simulink model "fft_dsp_lib"  (R2021a)
settings: Solver=VariableStepAuto  StartTime=0.0  StopTime=1  RelTol=1e-3
undefined symbols (not defined in the file): xc7vx485tffg1157
libraries: simulink x1, dspxfrm3 x1, vmcUtilities x1, dspsrcs4 x1, aieUtilities x1, aieDSP x1
settings Model: Creator=abehbood  LastModifiedBy=abehbood
settings SolverCC: AlgebraicLoopSolver=TrustRegion
settings DebuggingCC: SFMachineParentedDataDiag=warning
settings HardwareCC: ProdBitPerPointer=32  ProdBitPerSizeT=32  ProdBitPerPtrDiffT=32  ProdLargestAtomicFloat=None  ProdIntDivRoundTo=Undefined  ProdEndianess=Unspecified  ProdWordSize=32  ProdHWDeviceType=ASIC/FPGA->ASIC/FPGA  TargetBitPerLong=64  TargetBitPerPointer=64  TargetBitPerSizeT=64  TargetBitPerPtrDiffT=64  TargetLongLongMode=on  TargetIntDivRoundTo=Zero  TargetEndianess=LittleEndian  TargetWordSize=64  TargetHWDeviceType=Custom Processor->MATLAB Host Computer  ProdEqTarget=off

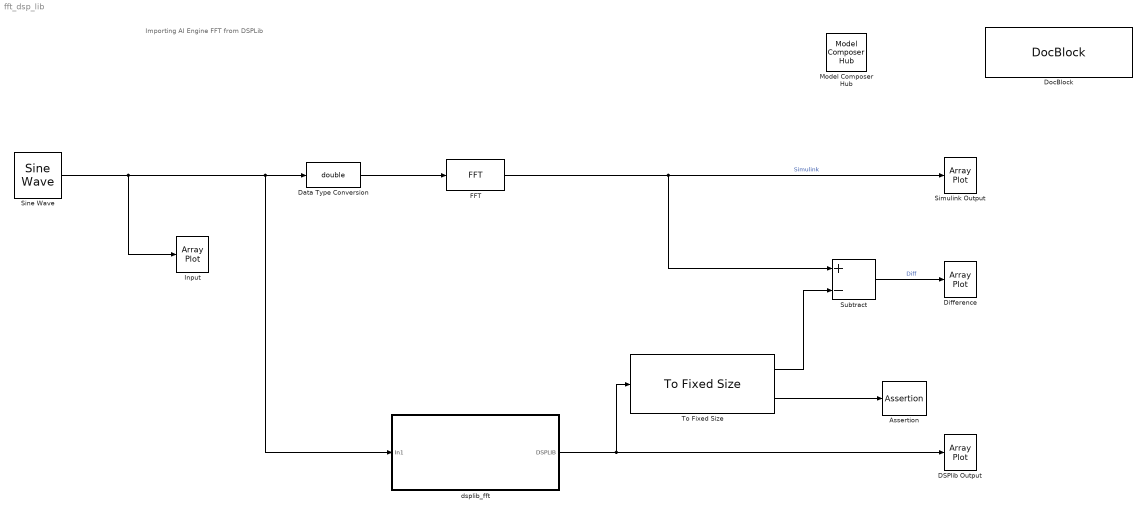
== system fft_dsp_lib ==
  note: Importing AI Engine FFT from DSPLib
  Assertion : Assertion
  DSPlib Output : ArrayPlot  WindowPosition=[34.000000,414.000000,816.000000,354.000000,]  Visible=on  AxesScaling=Manual  YLimits=[-23969.1,17302.1]  ShowLegend=on  DefaultConfigurationName=dsp.scopes.ArrayPlotBlockSpecification
  Data Type Conversion : DataTypeConversion  OutDataTypeStr=double
  Difference : ArrayPlot  WindowPosition=[4.000000,48.000000,780.000000,336.000000,]  Visible=on  AxesScaling=Manual  Title=Difference between AI Engine and Simulink  YLimits=[-461.936,415.69]  ShowLegend=on  DefaultConfigurationName=dsp.scopes.ArrayPlotBlockSpecification
  DocBlock : simulink/Model-Wide Utilities/DocBlock  DocumentType=Text  mask(DocBlock){}
      content=|
      | ///////////////////////////////////////////////////////////////////////////
      | // Copyright 2021 Xilinx
      | //
      | // Licensed under the Apache License, Version 2.0 (the "License");
      | // you may not use this file except in compliance with the License.
      | // You may obtain a copy of the License at
      | //
      | // http://www.apache.org/licenses/LICENSE-2.0
      | //
      | // Unless required by applicable law or agreed to in writing, software
      | // distributed under the License is distributed on an "AS IS" BASIS,
      | // WITHOUT WARRANTIES OR CONDITIONS OF ANY KIND, either express or implied.
      | // See the License for the specific language governing permissions and
      | // limitations under the License.
      | ///////////////////////////////////////////////////////////////////////////
      mask Display:
      | xmcDrawBlockIcon();
      | disp(['{\fontsize{10pt}(c) Copyright 2021' ' Xilinx, Inc.}\newline \newline '],'texmode','on');
      | disp('{\fontsize{10pt}Licensed under the Apache License 2.0}','texmode','on');
      | disp('\newline \newline \newline{\fontsize{10pt}Double Click for Copyright Notice}','texmode','on');
  FFT : dspxfrm3/FFT  FFTImplementation=Auto  CompMethod=Table lookup  TableOpt=NEW  TableOptActive=Speed  BitRevOrder=off  Normalize=off  InheritFFTLength=on  FFTLength=64  WrapInput=on  roundingMode=Floor  overflowMode=off  firstCoeffDataTypeStr=Inherit: Same word length as input  firstCoeffLastDataTypeStr=Inherit: Same word length as input  outputMin=[]  outputMax=[]
  Input : ArrayPlot  WindowPosition=[913.000000,42.000000,864.000000,406.000000,]  Visible=on  AxesScaling=Manual  YLimits=[-160,160]  ShowLegend=on  DefaultConfigurationName=dsp.scopes.ArrayPlotBlockSpecification
  Model Composer Hub : vmcUtilities/Model Composer Hub  CodeGeneration=off  SubsystemName=dsplib_fft  TargetDirectory=./code  ExportType=AI Engines  IpVendor=xilinx.com  IpLibrary=hls  IpVersion=1.0  IpHWLanguage=Verilog  AieCompilerOptions={}  CreateTestbench=on  TestbenchStackSize=10  RunAieSim=on  AieSimTimeout=50000  RunAieSimProfiling=off  LaunchVitisAnalyzer=off  PlotOutput=off  RunX86Sim=off  X86SimTimeout=10  GenHwImage=off  PlatformType=Not Specified  HwSystemType=Baremetal  HwValidationTarget=hw  ProjDevice=xc7vx485tffg1157-1  ProjDevicePart=xc7vx485tffg1157-1  SamplePeriod=-1  ClockFrequency=200  DataPathParallelism=1  xilinxfamily=Kintex7  part=xc7k325t  speed=-3  package=fbg676  directory=./netlist  testbench=off  incr_netlist=off  synthesis_tool=Vivado  clock_wrapper=Clock Enables  dbl_ovrd=According to Block Masks  dcm_input_clock_period=10  sysclk_period=10  simulink_period=1  eval_field=0
  Simulink Output : ArrayPlot  WindowPosition=[963.000000,389.000000,850.000000,415.000000,]  Visible=on  AxesScaling=Manual  YLimits=[-23966.4,17294.7]  ShowLegend=on  DefaultConfigurationName=dsp.scopes.ArrayPlotBlockSpecification
  Sine Wave : dspsrcs4/Sine Wave  Amplitude=64  Frequency=200  Phase=0  SampleMode=Discrete  OutComplex=Complex  CompMethod=Table lookup  TableSize=Speed  SampleTime=1/1000  SamplesPerFrame=512  ResetState=Restart at time zero  OutputFrames=off  dataType=Fixed-point  wordLen=16  udDataType=sfix(16)  fracBitsMode=User-defined  numFracBits=0  OutDataTypeStr=fixdt(1,16,0)  LastOutDataTypeStr=fixdt(1,16,0)
  Subtract : Sum  Inputs=+-
  To Fixed Size : aieUtilities/To Fixed Size  OutputSize=512  CopyMethod=Buffer samples to form output  HasStatusOutput=on
  dsplib_fft : Subsystem
  wires:
  FFT/1 -> Subtract/1, Simulink Output/1  "Simulink"
  Subtract/1 -> Difference/1  "Diff"
  To Fixed Size/1 -> Subtract/2
  To Fixed Size/2 -> Assertion/1
  Sine Wave/1 -> Input/1, dsplib_fft/1(In1), Data Type Conversion/1
  Data Type Conversion/1 -> FFT/1
  dsplib_fft/1(DSPLIB) -> To Fixed Size/1, DSPlib Output/1

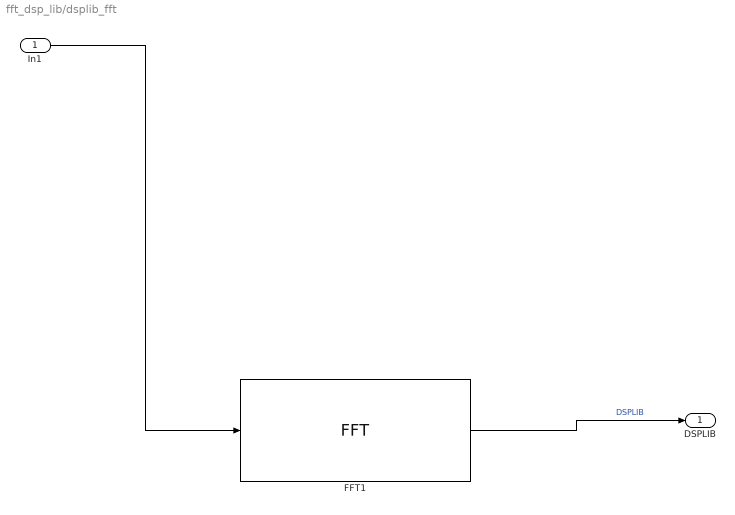
== system fft_dsp_lib/dsplib_fft ==
  In1 : Inport
  FFT1 : aieDSP/FFT  data_type=cint16  point_size=512  input_window_size=512  shift_val=0  input_sampling_rate=200  use_casc_length=on  casc_length=1  spec=meta_data_hl_fft.json
  DSPLIB : Outport
  wires:
  FFT1/1 -> DSPLIB/1  "DSPLIB"
  In1/1 -> FFT1/1
